simulink model "Relay_Pilot_Concept"  (R2020a)
settings: Solver=FixedStepAuto  StartTime=0.0  StopTime=10.0  FixedStep=0.0001  RelTol=1e-3
undefined symbols (not defined in the file): DiscIntNeverNeededParam
settings Model: Creator=BEDNASA  LastModifiedBy=BEDNASA

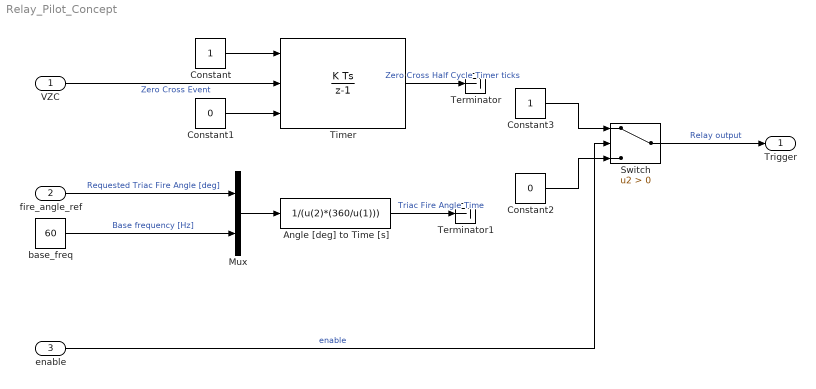
== system Relay_Pilot_Concept ==
  VZC : Inport
  fire_angle_ref : Inport  Port=2
  enable : Inport  Port=3
  Angle [deg] to Time [s] : Fcn  Expr=1/(u(2)*(360/u(1)))
  Constant : Constant
  Constant1 : Constant  Value=0
  Constant2 : Constant  Value=0  OutDataTypeStr=boolean
  Constant3 : Constant  OutDataTypeStr=boolean
  Mux : Mux  Inputs=2
  Switch : Switch  Criteria=u2 > Threshold
  Terminator : Terminator
  Terminator1 : Terminator
  Timer : DiscreteIntegrator  ExternalReset=either  InitialConditionSource=external  SampleTime=-1  ICPrevOutput=DiscIntNeverNeededParam  ICPrevScaledInput=DiscIntNeverNeededParam
  base_freq : Constant  Value=60  SampleTime=-1
  Trigger : Outport
  wires:
  Mux/1 -> Angle [deg] to Time [s]/1
  base_freq/1 -> Mux/2  "Base frequency [Hz]"
  fire_angle_ref/1 -> Mux/1  "Requested Triac Fire Angle [deg]"
  Constant/1 -> Timer/1
  Constant1/1 -> Timer/3
  VZC/1 -> Timer/2  "Zero Cross Event"
  Switch/1 -> Trigger/1  "Relay output"
  Constant2/1 -> Switch/3
  Constant3/1 -> Switch/1
  enable/1 -> Switch/2  "enable"
  Timer/1 -> Terminator/1  "Zero Cross Half Cycle Timer ticks"
  Angle [deg] to Time [s]/1 -> Terminator1/1  "Triac Fire Angle Time"
